simulink model "testFIR4"  (Simulink 7.0)
settings: Solver=FixedStepDiscrete  StartTime=0.0  StopTime=1000.0  RelTol=1e-3
undefined symbols (not defined in the file or in its folder): dfilt
libraries: dsparch4 x3
settings Model: Creator=epokh  LastModifiedBy=epokh
settings DebuggingCC: SolverPrmCheckMsg=none

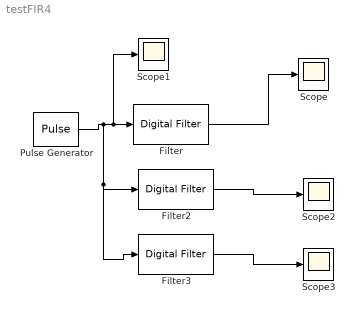
== system testFIR4 ==
  Filter : dsparch4/Digital Filter  Tag=BlockMethodSubSystem  DialogController=dspdialog.DigitalFilter  DialogControllerArgs=DataTag0  TypePopup=FIR (all zeros)  IIRFiltStruct=Direct form II transposed  AllPoleFiltStruct=Direct form  FIRFiltStruct=Direct form  CoeffSource=Specify via dialog  NumCoeffs=[-0.00504815393570616 0.318231068647215 0.505051444085258 0.318231068647215 -0.00504815393570616]  DenCoeffs=[1 0.1]  BiQuadCoeffs=[1 0.3 0.4 1 0.1 0.2]  LatticeCoeffs=[0.2 0.4]  denIgnore=on  FiltPerSampPopup=One filter per frame  IC=0  ICnum=0  ICden=0  roundingMode=Floor  overflowMode=off  ScaleValues=1  scaleValueFracLength=14  stageInFracLength=15  stageOutFracLength=15  FilterSource=Specify via dialog  dfiltObjectName=dfilt.dffir([1 2 1])
  Filter2 : dsparch4/Digital Filter  Tag=BlockMethodSubSystem  DialogController=dspdialog.DigitalFilter  DialogControllerArgs=DataTag1  TypePopup=IIR (poles & zeros)  IIRFiltStruct=Biquad direct form II (SOS)  AllPoleFiltStruct=Direct form  FIRFiltStruct=Direct form  CoeffSource=Specify via dialog  NumCoeffs=[1 2]  DenCoeffs=[1 0.1]  BiQuadCoeffs=[1 -6.82842712474619 1 1 0 0;0.25 0.5 0.25 1 0 0]  LatticeCoeffs=[0.2 0.4]  denIgnore=on  FiltPerSampPopup=One filter per frame  IC=0  ICnum=0  ICden=0  roundingMode=Floor  overflowMode=off  ScaleValues=[-0.207106781186548;1;1]  scaleValueFracLength=14  stageInFracLength=15  stageOutFracLength=15  FilterSource=Specify via dialog  dfiltObjectName=dfilt.dffir([1 2 1])
  Filter3 : dsparch4/Digital Filter  Tag=BlockMethodSubSystem  DialogController=dspdialog.DigitalFilter  DialogControllerArgs=DataTag2  TypePopup=IIR (poles & zeros)  IIRFiltStruct=Biquad direct form II (SOS)  AllPoleFiltStruct=Direct form  FIRFiltStruct=Direct form  CoeffSource=Specify via dialog  NumCoeffs=[1 2]  DenCoeffs=[1 0.1]  BiQuadCoeffs=[1 6.59045335781159 0.999999999999999 1 0 0;0.25 0.5 0.25 1 0 0;0.25 0.5 0.25 1 0 0;0.25 0.5 0.25 1 0 0]  LatticeCoeffs=[0.2 0.4]  denIgnore=on  FiltPerSampPopup=One filter per frame  IC=0  ICnum=0  ICden=0  roundingMode=Floor  overflowMode=off  ScaleValues=[0.116408291663753;1;1;1;1]  scaleValueFracLength=14  stageInFracLength=15  stageOutFracLength=15  FilterSource=Specify via dialog  dfiltObjectName=dfilt.dffir([1 2 1])
  Pulse Generator : DiscretePulseGenerator  Period=100  PulseWidth=10
  Scope{,1..3} (4 alike) : Scope
      Scope2 settings: SaveName=ScopeData2
      Scope3 settings: SaveName=ScopeData3
  wires:
  Pulse Generator/1 -> Filter/1, Scope1/1, Filter2/1, Filter3/1
  Filter/1 -> Scope/1
  Filter2/1 -> Scope2/1
  Filter3/1 -> Scope3/1
